simulink model "Exe3"  (R2023b)
settings: Solver=VariableStepAuto  StartTime=0.0  StopTime=1  RelTol=1e-3
undefined symbols (not defined in the file): designMultirateFIR
libraries: dspindex x4, dspmlti4 x4, dspstat3 x3
settings Model: PauseTimes=0.01  SnapshotInterval=1  PacingRate=1.100000  Creator=Fartash  LastModifiedBy=Fartash

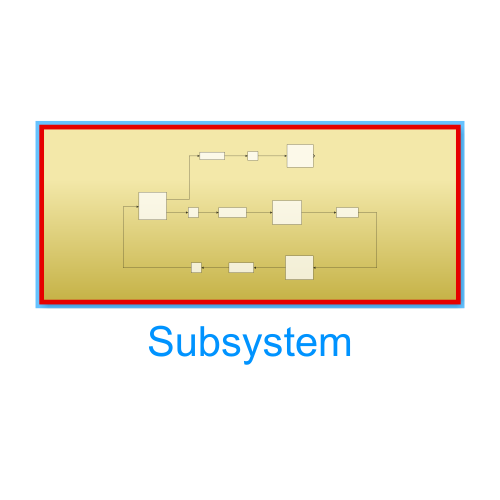
[thumbnail: Simulink's stored preview of the top-level diagram]
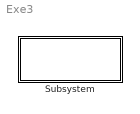
== system Exe3 ==
  Subsystem : Subsystem

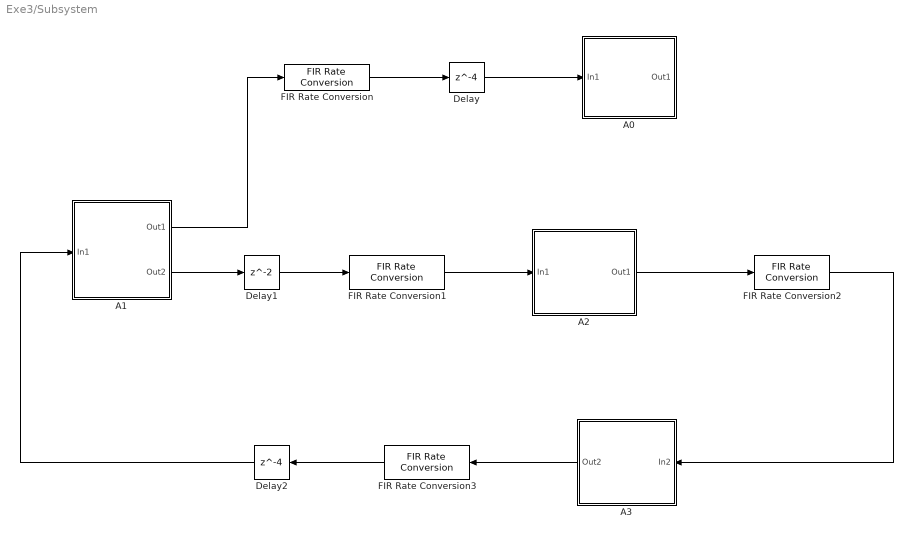
== system Exe3/Subsystem ==
  A0 : Subsystem
  A1 : Subsystem
  A2 : Subsystem
  A3 : Subsystem
  Delay : Delay  DelayLength=4
  Delay1 : Delay
  Delay2 : Delay  DelayLength=4
  FIR Rate Conversion : dspmlti4/FIR Rate Conversion  FilterSource=Auto  L=3  h=designMultirateFIR(3,2)  M=2  FilterObject=FRC  rateMode=Enforce single-rate processing  AllowArbitraryInputLength=off  roundingMode=Floor  overflowMode=off  firstCoeffDataTypeStr=Inherit: Same word length as input  firstCoeffMin=[]  firstCoeffMax=[]  firstCoeffLastDataTypeStr=Inherit: Same word length as input  outputDataTypeStr=Inherit: Same as accumulator  outputMin=[]  outputMax=[]  outputLastDataTypeStr=Inherit: Same as accumulator
  FIR Rate Conversion1 : dspmlti4/FIR Rate Conversion  FilterSource=Auto  L=3  h=designMultirateFIR(3,2)  M=1  FilterObject=FRC  rateMode=Enforce single-rate processing  AllowArbitraryInputLength=off  roundingMode=Floor  overflowMode=off  firstCoeffDataTypeStr=Inherit: Same word length as input  firstCoeffMin=[]  firstCoeffMax=[]  firstCoeffLastDataTypeStr=Inherit: Same word length as input  outputDataTypeStr=Inherit: Same as accumulator  outputMin=[]  outputMax=[]  outputLastDataTypeStr=Inherit: Same as accumulator
  FIR Rate Conversion2 : dspmlti4/FIR Rate Conversion  FilterSource=Auto  L=4  h=designMultirateFIR(3,2)  M=1  FilterObject=FRC  rateMode=Enforce single-rate processing  AllowArbitraryInputLength=off  roundingMode=Floor  overflowMode=off  firstCoeffDataTypeStr=Inherit: Same word length as input  firstCoeffMin=[]  firstCoeffMax=[]  firstCoeffLastDataTypeStr=Inherit: Same word length as input  outputDataTypeStr=Inherit: Same as accumulator  outputMin=[]  outputMax=[]  outputLastDataTypeStr=Inherit: Same as accumulator
  FIR Rate Conversion3 : dspmlti4/FIR Rate Conversion  FilterSource=Auto  L=4  h=designMultirateFIR(3,2)  M=3  FilterObject=FRC  rateMode=Enforce single-rate processing  AllowArbitraryInputLength=off  roundingMode=Floor  overflowMode=off  firstCoeffDataTypeStr=Inherit: Same word length as input  firstCoeffMin=[]  firstCoeffMax=[]  firstCoeffLastDataTypeStr=Inherit: Same word length as input  outputDataTypeStr=Inherit: Same as accumulator  outputMin=[]  outputMax=[]  outputLastDataTypeStr=Inherit: Same as accumulator
  wires:
  FIR Rate Conversion2/1 -> A3/1(In2)
  A2/1(Out1) -> FIR Rate Conversion2/1
  FIR Rate Conversion1/1 -> A2/1(In1)
  A1/1(Out1) -> FIR Rate Conversion/1
  A3/1(Out2) -> FIR Rate Conversion3/1
  FIR Rate Conversion3/1 -> Delay2/1
  FIR Rate Conversion/1 -> Delay/1
  Delay1/1 -> FIR Rate Conversion1/1
  A1/2(Out2) -> Delay1/1
  Delay2/1 -> A1/1(In1)
  Delay/1 -> A0/1(In1)

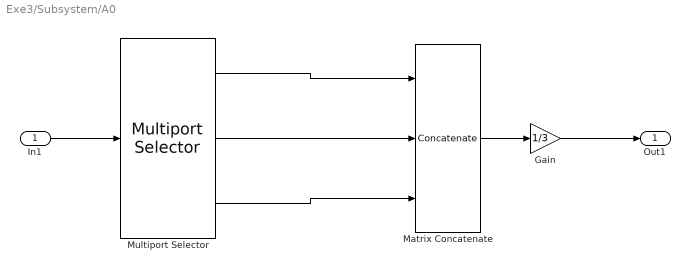
== system Exe3/Subsystem/A0 ==
  In1 : Inport
  Gain : Gain  Gain=1/3
  Matrix Concatenate : Concatenate  NumInputs=3  ConcatenateDimension=2
  Multiport Selector : dspindex/Multiport Selector  rowsOrCols=Rows  idxCellArray={1,2,3}  idxErrMode=Clip Index
      settings: LibrarySourceBlock=|
      | dsphdlsupportsigmgmt/Multiport
      | Selector
  Out1 : Outport
  wires:
  In1/1 -> Multiport Selector/1
  Gain/1 -> Out1/1
  Multiport Selector/1 -> Matrix Concatenate/1
  Multiport Selector/2 -> Matrix Concatenate/2
  Multiport Selector/3 -> Matrix Concatenate/3
  Matrix Concatenate/1 -> Gain/1

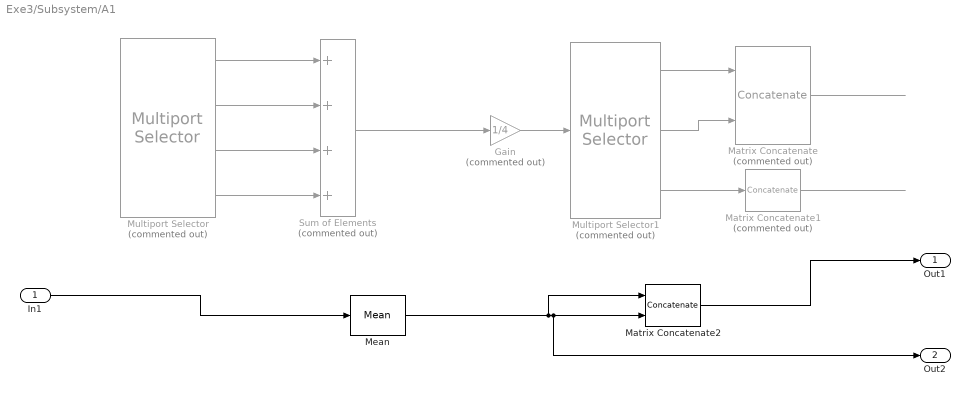
== system Exe3/Subsystem/A1 ==
  In1 : Inport
  Gain : Gain  Commented=on  Gain=1/4
  Matrix Concatenate : Concatenate  Commented=on  ConcatenateDimension=2
  Matrix Concatenate1 : Concatenate  Commented=on  NumInputs=1  ConcatenateDimension=2
  Matrix Concatenate2 : Concatenate  ConcatenateDimension=2
  Mean : dspstat3/Mean  run=off  InputProcessing=Columns as channels (frame based)  reset_popup=None  directionMode=Each column  dimension=1  roiEnable=off  roiType=Rectangles  roiPortion=Entire ROI  roiOutput=Individual statistics for each ROI  roiFlag=off  roundingMode=Floor  overflowMode=off  outputDataTypeStr=Inherit: Same as accumulator  outputMin=[]  outputMax=[]  outputLastDataTypeStr=Inherit: Same as accumulator
  Multiport Selector : dspindex/Multiport Selector  Commented=on  rowsOrCols=Rows  idxCellArray={ 1,2,3,4 }  idxErrMode=Clip Index
      settings: LibrarySourceBlock=|
      | dsphdlsupportsigmgmt/Multiport
      | Selector
  Multiport Selector1 : dspindex/Multiport Selector  Commented=on  rowsOrCols=Rows  idxCellArray={1,2,3}  idxErrMode=Clip Index
      settings: LibrarySourceBlock=|
      | dsphdlsupportsigmgmt/Multiport
      | Selector
  Sum of Elements : Sum  Commented=on  Inputs=++++
  Out1 : Outport
  Out2 : Outport  Port=2
  wires:
  Multiport Selector1/3 -> Matrix Concatenate1/1
  Sum of Elements/1 -> Gain/1
  ? -> Multiport Selector/1
  Multiport Selector/4 -> Sum of Elements/4
  Multiport Selector1/2 -> Matrix Concatenate/2
  Matrix Concatenate/1 -> ?
  Multiport Selector/3 -> Sum of Elements/3
  Matrix Concatenate1/1 -> ?
  Multiport Selector/2 -> Sum of Elements/2
  Multiport Selector/1 -> Sum of Elements/1
  Multiport Selector1/1 -> Matrix Concatenate/1
  Gain/1 -> Multiport Selector1/1
  In1/1 -> Mean/1
  Mean/1 -> Matrix Concatenate2/1, Out2/1, Matrix Concatenate2/2
  Matrix Concatenate2/1 -> Out1/1

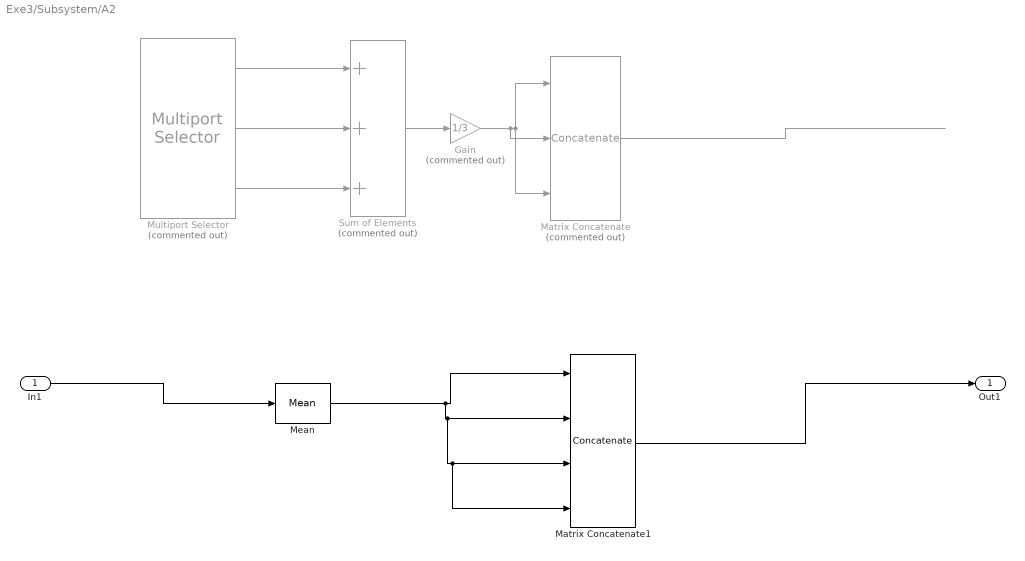
== system Exe3/Subsystem/A2 ==
  In1 : Inport
  Gain : Gain  Commented=on  Gain=1/3
  Matrix Concatenate : Concatenate  Commented=on  NumInputs=3  ConcatenateDimension=2
  Matrix Concatenate1 : Concatenate  NumInputs=4  ConcatenateDimension=2
  Mean : dspstat3/Mean  run=off  InputProcessing=Columns as channels (frame based)  reset_popup=None  directionMode=Each column  dimension=1  roiEnable=off  roiType=Rectangles  roiPortion=Entire ROI  roiOutput=Individual statistics for each ROI  roiFlag=off  roundingMode=Floor  overflowMode=off  outputDataTypeStr=Inherit: Same as accumulator  outputMin=[]  outputMax=[]  outputLastDataTypeStr=Inherit: Same as accumulator
  Multiport Selector : dspindex/Multiport Selector  Commented=on  rowsOrCols=Rows  idxCellArray={ 1,2,3}  idxErrMode=Clip Index
      settings: LibrarySourceBlock=|
      | dsphdlsupportsigmgmt/Multiport
      | Selector
  Sum of Elements : Sum  Commented=on  Inputs=+++
  Out1 : Outport
  wires:
  Gain/1 -> Matrix Concatenate/3, Matrix Concatenate/1, Matrix Concatenate/2
  Multiport Selector/2 -> Sum of Elements/2
  Multiport Selector/1 -> Sum of Elements/1
  Sum of Elements/1 -> Gain/1
  Multiport Selector/3 -> Sum of Elements/3
  Matrix Concatenate/1 -> ?
  ? -> Multiport Selector/1
  In1/1 -> Mean/1
  Mean/1 -> Matrix Concatenate1/4, Matrix Concatenate1/3, Matrix Concatenate1/2, Matrix Concatenate1/1
  Matrix Concatenate1/1 -> Out1/1

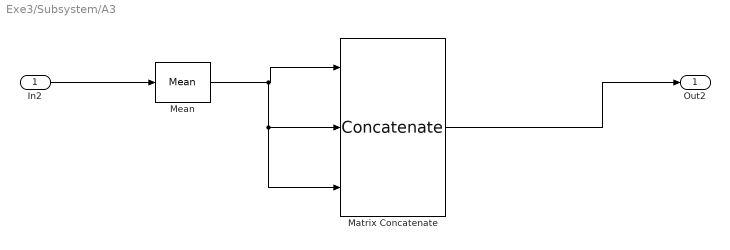
== system Exe3/Subsystem/A3 ==
  In2 : Inport
  Matrix Concatenate : Concatenate  NumInputs=3  ConcatenateDimension=2
  Mean : dspstat3/Mean  run=off  InputProcessing=Columns as channels (frame based)  reset_popup=None  directionMode=Each column  dimension=1  roiEnable=off  roiType=Rectangles  roiPortion=Entire ROI  roiOutput=Individual statistics for each ROI  roiFlag=off  roundingMode=Floor  overflowMode=off  outputDataTypeStr=Inherit: Same as accumulator  outputMin=[]  outputMax=[]  outputLastDataTypeStr=Inherit: Same as accumulator
  Out2 : Outport
  wires:
  In2/1 -> Mean/1
  Matrix Concatenate/1 -> Out2/1
  Mean/1 -> Matrix Concatenate/3, Matrix Concatenate/2, Matrix Concatenate/1
